simulink model "testing_model"  (R2024a)
settings: Solver=VariableStepAuto  StartTime=0.0  StopTime=30  RelTol=1e-3
values from neighbouring files (symbols this model uses):
  telescope0 = 4    [enviroment_setup.m]
  thetaList0 = [0, 0, 0, 0, 0]'    [enviroment_setup.m]
settings Model: Creator=larso  LastModifiedBy=larso

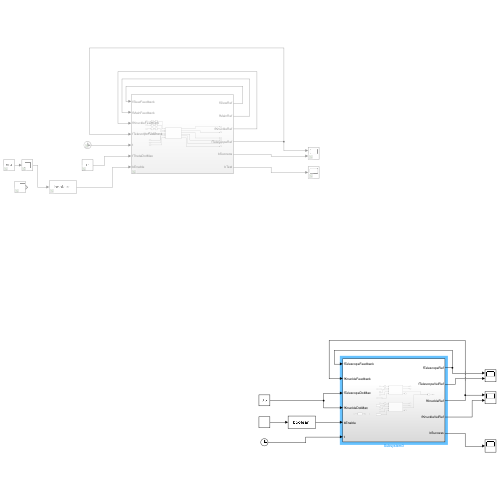
[thumbnail: Simulink's stored preview of the top-level diagram]
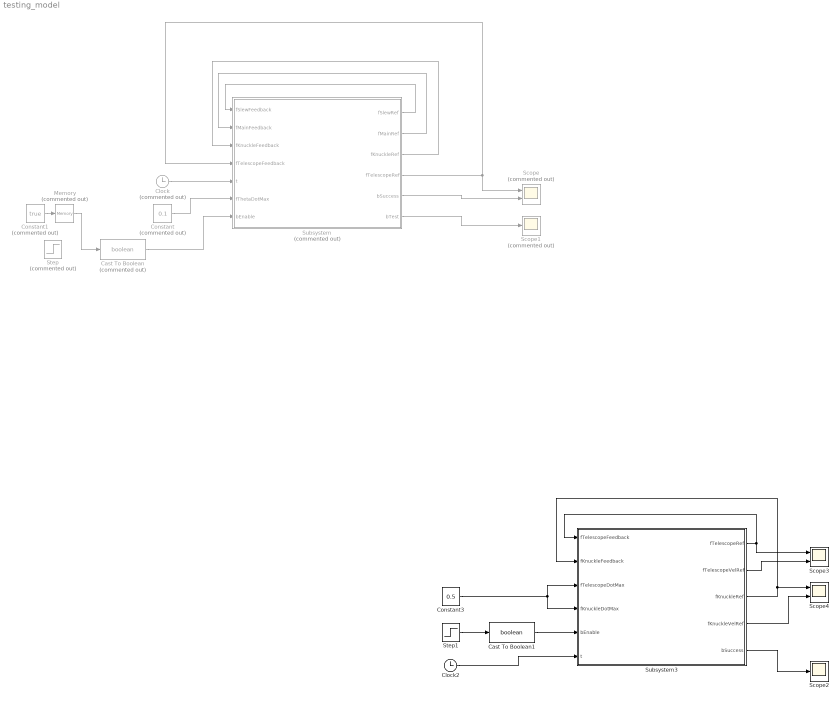
== system testing_model ==
  Cast To Boolean : DataTypeConversion  Commented=on  OutDataTypeStr=boolean  SaturateOnIntegerOverflow=off  RndMeth=Floor
  Cast To Boolean1 : DataTypeConversion  OutDataTypeStr=boolean  SaturateOnIntegerOverflow=off  RndMeth=Floor
  Clock : Clock  Commented=on
  Clock2 : Clock
  Constant : Constant  Commented=on  Value=0.1
  Constant1 : Constant  Commented=on  Value=true
  Constant3 : Constant  Value=0.5
  Memory : Memory  Commented=on  InitialCondition=false
  Scope : Scope  Commented=on  NumInputPorts=2
  Scope1 : Scope  Commented=on
  Scope2 : Scope
  Scope3 : Scope  NumInputPorts=2
  Scope4 : Scope  NumInputPorts=2
  Step : Step  Commented=on  SampleTime=0
  Step1 : Step  SampleTime=0
  Subsystem : Subsystem  Commented=on
  Subsystem3 : Subsystem
  wires:
  Subsystem/1(fSlewRef) -> Subsystem/1(fSlewFeedback)
  Subsystem/2(fMainRef) -> Subsystem/2(fMainFeedback)
  Subsystem/3(fKnuckleRef) -> Subsystem/3(fKnuckleFeedback)
  Subsystem/4(fTelescopeRef) -> Scope/1, Subsystem/4(fTelescopeFeedback)
  Constant1/1 -> Memory/1
  Constant/1 -> Subsystem/6(fThetaDotMax)
  Clock/1 -> Subsystem/5(t)
  Cast To Boolean/1 -> Subsystem/7(bEnable)
  Subsystem/5(bSuccess) -> Scope/2
  Memory/1 -> Cast To Boolean/1
  Subsystem/6(bTest) -> Scope1/1
  Step1/1 -> Cast To Boolean1/1
  Subsystem3/1(fTelescopeRef) -> Scope3/1, Subsystem3/1(fTelescopeFeedback)
  Clock2/1 -> Subsystem3/6(t)
  Cast To Boolean1/1 -> Subsystem3/5(bEnable)
  Subsystem3/5(bSuccess) -> Scope2/1
  Subsystem3/2(fTelescopeVelRef) -> Scope3/2
  Subsystem3/3(fKnuckleRef) -> Subsystem3/2(fKnuckleFeedback), Scope4/1
  Subsystem3/4(fKnuckleVelRef) -> Scope4/2
  Constant3/1 -> Subsystem3/3(fTelescopeDotMax), Subsystem3/4(fKnuckleDotMax)

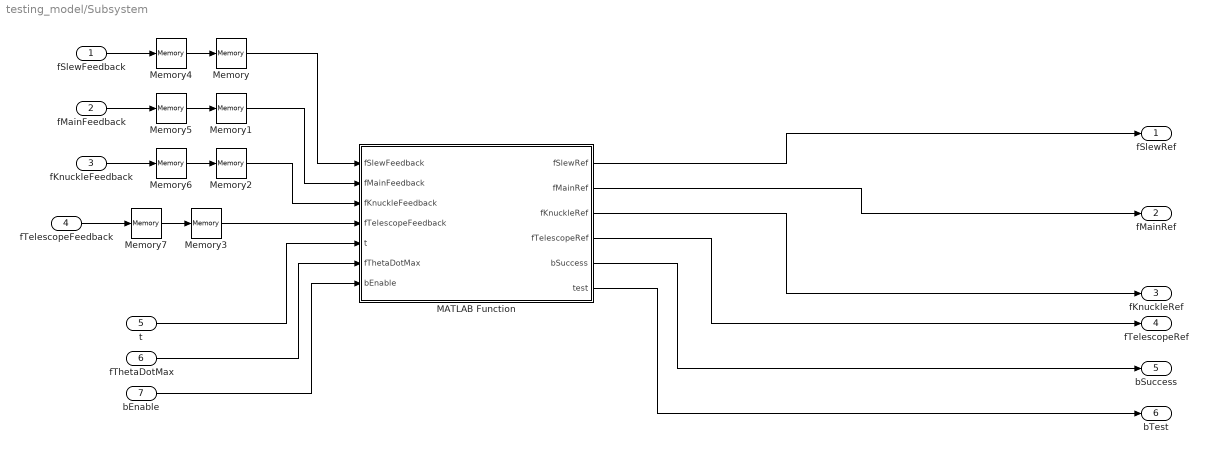
== system testing_model/Subsystem ==
  fSlewFeedback : Inport
  fMainFeedback : Inport  Port=2
  fKnuckleFeedback : Inport  Port=3
  fTelescopeFeedback : Inport  Port=4
  t : Inport  Port=5
  fThetaDotMax : Inport  Port=6
  bEnable : Inport  Port=7
  MATLAB Function : MATLAB Function  TreatAsAtomicUnit=on
  Memory : Memory  InitialCondition=thetaList0(1)
  Memory1 : Memory  InitialCondition=thetaList0(2)
  Memory2 : Memory  InitialCondition=thetaList0(3)
  Memory3 : Memory  InitialCondition=telescope0
  Memory4 : Memory  InitialCondition=thetaList0(1)
  Memory5 : Memory  InitialCondition=thetaList0(2)
  Memory6 : Memory  InitialCondition=thetaList0(3)
  Memory7 : Memory  InitialCondition=telescope0
  fSlewRef : Outport
  fMainRef : Outport  Port=2
  fKnuckleRef : Outport  Port=3
  fTelescopeRef : Outport  Port=4
  bSuccess : Outport  Port=5
  bTest : Outport  Port=6
  wires:
  MATLAB Function/4(fTelescopeRef) -> fTelescopeRef/1
  MATLAB Function/2(fMainRef) -> fMainRef/1
  fMainFeedback/1 -> Memory5/1
  fSlewFeedback/1 -> Memory4/1
  fKnuckleFeedback/1 -> Memory6/1
  MATLAB Function/5(bSuccess) -> bSuccess/1
  t/1 -> MATLAB Function/5(t)
  MATLAB Function/1(fSlewRef) -> fSlewRef/1
  MATLAB Function/3(fKnuckleRef) -> fKnuckleRef/1
  fThetaDotMax/1 -> MATLAB Function/6(fThetaDotMax)
  bEnable/1 -> MATLAB Function/7(bEnable)
  fTelescopeFeedback/1 -> Memory7/1
  Memory/1 -> MATLAB Function/1(fSlewFeedback)
  Memory1/1 -> MATLAB Function/2(fMainFeedback)
  Memory2/1 -> MATLAB Function/3(fKnuckleFeedback)
  Memory3/1 -> MATLAB Function/4(fTelescopeFeedback)
  Memory7/1 -> Memory3/1
  Memory4/1 -> Memory/1
  Memory5/1 -> Memory1/1
  Memory6/1 -> Memory2/1
  MATLAB Function/6(test) -> bTest/1

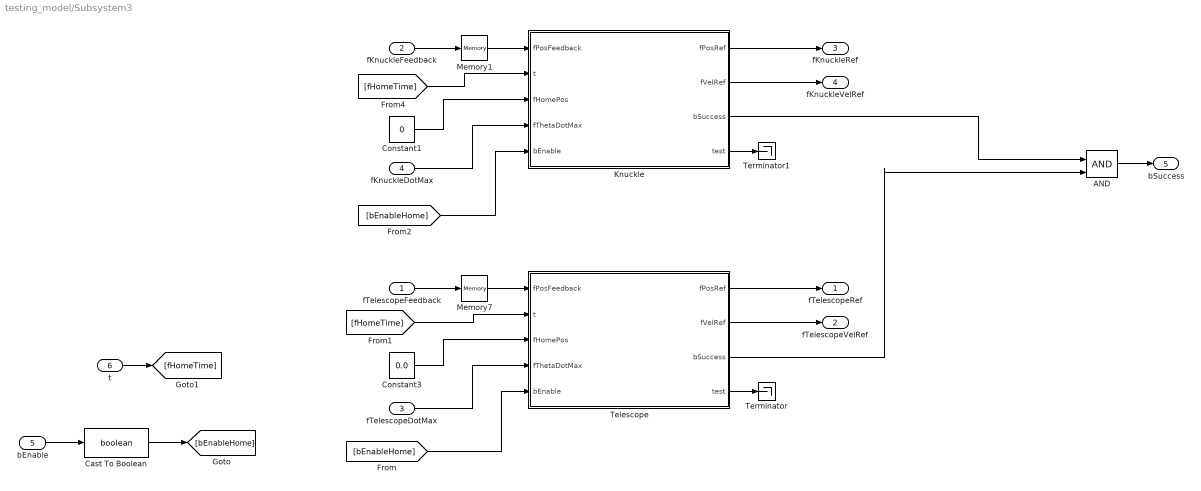
== system testing_model/Subsystem3 ==
  fTelescopeFeedback : Inport
  fKnuckleFeedback : Inport  Port=2
  fTelescopeDotMax : Inport  Port=3
  fKnuckleDotMax : Inport  Port=4
  bEnable : Inport  Port=5
  t : Inport  Port=6
  AND : Logic  IconShape=distinctive  AllPortsSameDT=off  OutDataTypeStr=boolean
  Cast To Boolean : DataTypeConversion  OutDataTypeStr=boolean  SaturateOnIntegerOverflow=off  RndMeth=Floor
  Constant1 : Constant  Value=0
  Constant3 : Constant  Value=0.0
  Knuckle : MATLAB Function  TreatAsAtomicUnit=on
  Memory1 : Memory  InitialCondition=thetaList0(3)
  Memory7 : Memory  InitialCondition=telescope0
  Telescope : MATLAB Function  TreatAsAtomicUnit=on
  Terminator : Terminator
  Terminator1 : Terminator
  fTelescopeRef : Outport
  fTelescopeVelRef : Outport  Port=2
  fKnuckleRef : Outport  Port=3
  fKnuckleVelRef : Outport  Port=4
  bSuccess : Outport  Port=5
  wires:
  Telescope/1(fPosRef) -> fTelescopeRef/1
  Telescope/3(bSuccess) -> AND/2
  [fHomeTime] -> Telescope/2(t)
  fTelescopeDotMax/1 -> Telescope/4(fThetaDotMax)
  [bEnableHome] -> Telescope/5(bEnable)
  fTelescopeFeedback/1 -> Memory7/1
  Constant3/1 -> Telescope/3(fHomePos)
  Memory7/1 -> Telescope/1(fPosFeedback)
  Telescope/2(fVelRef) -> fTelescopeVelRef/1
  Telescope/4(test) -> Terminator/1
  Constant1/1 -> Knuckle/3(fHomePos)
  Knuckle/3(bSuccess) -> AND/1
  Knuckle/2(fVelRef) -> fKnuckleVelRef/1
  Memory1/1 -> Knuckle/1(fPosFeedback)
  Knuckle/4(test) -> Terminator1/1
  Knuckle/1(fPosRef) -> fKnuckleRef/1
  [bEnableHome] -> Knuckle/5(bEnable)
  fKnuckleDotMax/1 -> Knuckle/4(fThetaDotMax)
  [fHomeTime] -> Knuckle/2(t)
  fKnuckleFeedback/1 -> Memory1/1
  AND/1 -> bSuccess/1
  bEnable/1 -> Cast To Boolean/1
  t/1 -> [fHomeTime]
  Cast To Boolean/1 -> [bEnableHome]

== matlab function testing_model/Subsystem/MATLAB Function ==
  settings: updateMethod=DISCRETE
  data: fSlewFeedback input; fSlewRef output; fMainRef output; fKnuckleRef output; fTelescopeRef output; fMainFeedback input; fKnuckleFeedback input; fTelescopeFeedback input; t input; bSuccess output; fThetaDotMax input; bEnable input; test output
function [fSlewRef, fMainRef, fKnuckleRef, fTelescopeRef, bSuccess, test] = ...
                    goHome(fSlewFeedback, ...
                    fMainFeedback, ...
                    fKnuckleFeedback, ...
                    fTelescopeFeedback, ...
                    t,...
                    fThetaDotMax, ...
                    bEnable)
bSuccess = false;


%fSlewRef = 0;
%fMainRef = 0;
%fKnuckleRef = 0;
%fTelescopeRef = 0;

slewHomeTheta = 0.0;
mainHomeTheta = 0.0;
knuckleHomeTheta = 0.0;
telescopeHomeTheta = 2.0;


[fSlewRef, ~, bSlewDone, ~] = cosinePositionGenerator(fSlewFeedback, slewHomeTheta, fThetaDotMax, t, bEnable);
[fMainRef, ~, bMainDone, ~] = cosinePositionGenerator(fMainFeedback, mainHomeTheta, fThetaDotMax, t, bEnable);
[fKnuckleRef, ~, bKnuckleDone, ~] = cosinePositionGenerator(fKnuckleFeedback, knuckleHomeTheta, fThetaDotMax, t, bEnable);

[fTelescopeRef, ~, bTelescopeDone, test] = cosinePositionGenerator(fTelescopeFeedback, telescopeHomeTheta, fThetaDotMax, t, bEnable);

if (bSlewDone & bMainDone & bKnuckleDone & bTelescopeDone)
    bSuccess = true;
end



end

== matlab function testing_model/Subsystem3/Knuckle ==
  settings: updateMethod=DISCRETE
  data: fPosRef output; fVelRef output; fPosFeedback input; t input; fHomePos input; bSuccess output; fThetaDotMax input; bEnable input; test output
function [fPosRef, fVelRef, bSuccess, test] = goHomeKnuckle(fPosFeedback, ...
    t,...
    fHomePos,...
    fThetaDotMax, ...
    bEnable)

bSuccess = false;
fPosRef = 0.0;
fVelRef = 0.0;
test = false;




[fPosRef, fVelRef, bSuccess, test] = cosinePositionGenerator(fPosFeedback, fHomePos, fThetaDotMax, t, bEnable);



end

== matlab function testing_model/Subsystem3/Telescope ==
  settings: updateMethod=DISCRETE
  data: fPosRef output; fVelRef output; fPosFeedback input; t input; fHomePos input; bSuccess output; fThetaDotMax input; bEnable input; test output
function [fPosRef, fVelRef, bSuccess, test] = goHomeTelescope(fPosFeedback, ...
    t,...
    fHomePos,...
    fThetaDotMax, ...
    bEnable)

bSuccess = false;
fPosRef = 0.0;
fVelRef = 0.0;
test = false;


[fPosRef, fVelRef, bSuccess, test] = cosinePositionGenerator(fPosFeedback, fHomePos, fThetaDotMax, t, bEnable);



end
